simulink model "model_5_2"  (R2020a)
settings: Solver=VariableStepAuto  StartTime=0.0  StopTime=10.0  RelTol=1e-3
settings Model: Creator=Shadman  LastModifiedBy=Shadman

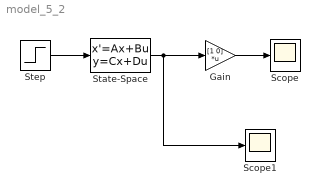
== system model_5_2 ==
  Gain : Gain  Gain=[1 0]  Multiplication=Matrix(K*u)
  Scope : Scope
  Scope1 : Scope
  State-Space : StateSpace  A=[0 1; -4 -2]  B=[0; 4]  C=[1 0; 0 1]  D=[0; 0]  InitialCondition=0
  Step : Step  Time=0  SampleTime=0
  wires:
  Step/1 -> State-Space/1
  State-Space/1 -> Scope1/1, Gain/1
  Gain/1 -> Scope/1
